simulink model "feedback_linearization_control"  (R2018b)
settings: Solver=VariableStepAuto  StartTime=0.0  StopTime=20  RelTol=1e-3
settings Model: Creator=Amirhossein  LastModifiedBy=Amirhossein

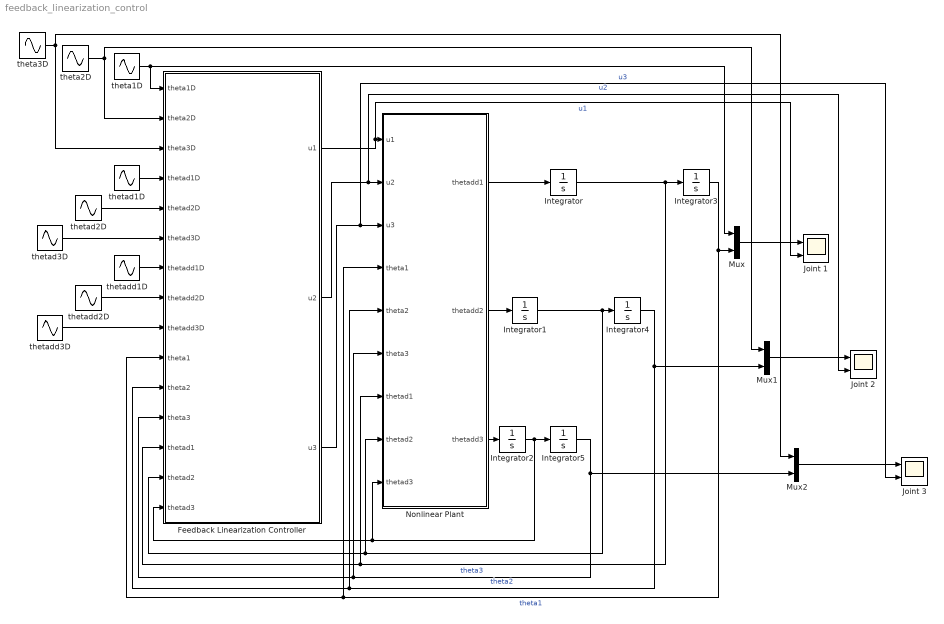
== system feedback_linearization_control ==
  Feedback Linearization Controller : MATLAB Function  TreatAsAtomicUnit=on
  Integrator{,1..5} (6 alike) : Integrator
  Joint 1 : Scope  NumInputPorts=2
  Joint 2 : Scope  NumInputPorts=2
  Joint 3 : Scope  NumInputPorts=2
  Mux : Mux  Inputs=2
  Mux1 : Mux  Inputs=2
  Mux2 : Mux  Inputs=2
  Nonlinear Plant : MATLAB Function  TreatAsAtomicUnit=on
  theta1D : Sin  SampleTime=0
  theta2D : Sin  Frequency=2  SampleTime=0
  theta3D : Sin  Frequency=3  SampleTime=0
  thetad1D : Sin  Phase=pi/2  SampleTime=0
  thetad2D : Sin  Amplitude=2  Frequency=2  Phase=pi/2  SampleTime=0
  thetad3D : Sin  Amplitude=3  Frequency=3  Phase=pi/2  SampleTime=0
  thetadd1D : Sin  Amplitude=-1  SampleTime=0
  thetadd2D : Sin  Amplitude=-4  Frequency=2  SampleTime=0
  thetadd3D : Sin  Amplitude=-9  Frequency=3  SampleTime=0
  wires:
  Integrator1/1 -> Integrator4/1, Feedback Linearization Controller/14(thetad2), Nonlinear Plant/8(thetad2)
  Integrator2/1 -> Feedback Linearization Controller/15(thetad3), Nonlinear Plant/9(thetad3), Integrator5/1
  Nonlinear Plant/1(thetadd1) -> Integrator/1
  Integrator/1 -> Feedback Linearization Controller/13(thetad1), Nonlinear Plant/7(thetad1), Integrator3/1
  Nonlinear Plant/2(thetadd2) -> Integrator1/1
  Nonlinear Plant/3(thetadd3) -> Integrator2/1
  Integrator3/1 -> Mux/2, Feedback Linearization Controller/10(theta1), Nonlinear Plant/4(theta1)  "theta1"
  Integrator4/1 -> Mux1/2, Feedback Linearization Controller/11(theta2), Nonlinear Plant/5(theta2)  "theta2"
  Feedback Linearization Controller/2(u2) -> Joint 2/2, Nonlinear Plant/2(u2)  "u2"
  Feedback Linearization Controller/1(u1) -> Joint 1/2, Nonlinear Plant/1(u1)  "u1"
  Feedback Linearization Controller/3(u3) -> Joint 3/2, Nonlinear Plant/3(u3)  "u3"
  Integrator5/1 -> Mux2/2, Feedback Linearization Controller/12(theta3), Nonlinear Plant/6(theta3)  "theta3"
  Mux1/1 -> Joint 2/1
  Mux2/1 -> Joint 3/1
  thetadd3D/1 -> Feedback Linearization Controller/9(thetadd3D)
  thetad1D/1 -> Feedback Linearization Controller/4(thetad1D)
  thetadd1D/1 -> Feedback Linearization Controller/7(thetadd1D)
  thetad3D/1 -> Feedback Linearization Controller/6(thetad3D)
  thetadd2D/1 -> Feedback Linearization Controller/8(thetadd2D)
  thetad2D/1 -> Feedback Linearization Controller/5(thetad2D)
  theta1D/1 -> Feedback Linearization Controller/1(theta1D), Mux/1
  theta2D/1 -> Mux1/1, Feedback Linearization Controller/2(theta2D)
  theta3D/1 -> Mux2/1, Feedback Linearization Controller/3(theta3D)
  Mux/1 -> Joint 1/1

== matlab function feedback_linearization_control/Feedback Linearization Controller ==
  data: theta1D input; theta2D input; u1 output; theta3D input; thetad1D input; thetad2D input; thetad3D input; thetadd1D input; thetadd2D input; thetadd3D input; theta1 input; theta2 input; theta3 input; thetad1 input; thetad2 input; thetad3 input; u2 output; u3 output
function [u1, u2, u3] = fcn(theta1D, theta2D, theta3D, thetad1D, thetad2D, thetad3D, thetadd1D, thetadd2D, thetadd3D, theta1, theta2, theta3, thetad1, thetad2, thetad3)

% lambda
lambda = 5;

thetaD = [theta1D; theta2D; theta3D];

thetadD = [thetad1D; thetad2D; thetad3D];

thetaddD = [thetadd1D; thetadd2D; thetadd3D];

% theta vector
theta = [theta1; theta2; theta3];

thetad = [thetad1; thetad2; thetad3];

e = theta - thetaD;

ed = thetad - thetadD;

%% model: the second model has been used

% the value of parameters
ma = 17.5e-3;
mc = 10.4e-3;
mbe = 0.2214;
mdf = 0.1106;
L1 = 13.97e-2;
L2 = 13.97e-2;
L3 = 0.325e-2;
L4 = 0.368e-2;
L5 = 0.527e-2;
g = 9.81;

% the elements of M matrix
m11 = ((0.5 * L1^2 + 0.125 * L2^2) * ma + (0.125 * L1^2 + 0.5 * L3^2) * mc) + 0.125 * L1^2 * (4*ma + mc) * cos(2*theta2) - 0.125 * (L2^2 * ma + 4 * L3^2 * mc) * cos(2*theta2) + 0.125 * (L2 * ma + L3 * mc) * cos(theta2) * sin(theta3);
m12 = 0;
m13 = 0;
m21 = m12;
m22 = L1^2 * (ma + 0.25 * mc);
m23 = -0.5 * L1 * (L2 * ma + L3 * mc) * sin(theta2 - theta3);
m31 = m13;
m32 = m23;
m33 = 0.25 * L2^2 * ma + L3^2 * mc;
% M matrix
M = [m11 m12 m13; m21 m22 m23; m31 m32 m33];

% the elements of V matrix
v11_1 = 0.25 * cos(theta3) * (2 * L1 * (L2 * ma + L3 * mc) * cos(theta2) + (L2^2 * ma + 4 * L3^2 * mc) * sin(theta3)) * thetad3;
v11 = 0.25 * (-2 * sin(theta2) * (L1^2 * (4 * ma + mc) * cos(theta2) + 2 * L1 * (L2 * ma + L3 * mc) * sin(theta3)) * thetad2) + v11_1;
v12 = -0.25 * (L1^2 * (4 * ma + mc) * sin(2 * theta2) + 2 * L1 * (L2 * ma + L3 * mc) * sin(theta2) * sin(theta3)) * thetad1;
v13 = -0.125 * (-4 * L1 * (L2 * ma + L3 * mc) * cos(theta2) * cos(theta3) - (L2^2 * ma + 4 * L3^2 * mc) * sin(2 * theta3)) * thetad1;
v21 = -v12;
v22 = 0;
v23 = 0.5 * L1 * (L2 * ma + L3 * mc) * cos(theta2 - theta3) * thetad3;
v31 = -v13;
v32 = 0.5 * L1 * (L2 * ma + L3 * mc) * cos(theta2 - theta3) * thetad2;
v33 = 0;
% V matrix
V = [v11 v12 v13; v21 v22 v23; v31 v32 v33];

% the elements of N vector
n1 = 0;
n2 = g * (L1 * (ma + 0.5 * mc) + L5 * mbe) * cos(theta2);
n3 = g * (0.5 * L2 * ma + L3 * mc - L4 * mdf ) * sin(theta3);
% N vector
N = [n1; n2; n3];

%%

W = thetaddD - 2 * lambda * ed - lambda^2 * e;

% U vector
U = M * W + V * thetad + N;

u1 = U(1);
u2 = U(2);
u3 = U(3);

== matlab function feedback_linearization_control/Nonlinear Plant ==
  data: u1 input; u2 input; thetadd1 output; u3 input; theta1 input; theta2 input; theta3 input; thetad1 input; thetad2 input; thetad3 input; thetadd2 output; thetadd3 output
function [thetadd1, thetadd2, thetadd3] = fcn(u1, u2, u3, theta1, theta2, theta3, thetad1, thetad2, thetad3)

% theta vector
thetad = [thetad1; thetad2; thetad3];

%% model: the second model has been used

% the value of parameters
ma = 17.5e-3;
mc = 10.4e-3;
mbe = 0.2214;
mdf = 0.1106;
L1 = 13.97e-2;
L2 = 13.97e-2;
L3 = 0.325e-2;
L4 = 0.368e-2;
L5 = 0.527e-2;
g = 9.81;

% the elements of M matrix
m11 = ((0.5 * L1^2 + 0.125 * L2^2) * ma + (0.125 * L1^2 + 0.5 * L3^2) * mc) + 0.125 * L1^2 * (4*ma + mc) * cos(2*theta2) - 0.125 * (L2^2 * ma + 4 * L3^2 * mc) * cos(2*theta2) + 0.125 * (L2 * ma + L3 * mc) * cos(theta2) * sin(theta3);
m12 = 0;
m13 = 0;
m21 = m12;
m22 = L1^2 * (ma + 0.25 * mc);
m23 = -0.5 * L1 * (L2 * ma + L3 * mc) * sin(theta2 - theta3);
m31 = m13;
m32 = m23;
m33 = 0.25 * L2^2 * ma + L3^2 * mc;
% M matrix
M = [m11 m12 m13; m21 m22 m23; m31 m32 m33];

% the elements of V matrix
v11_1 = 0.25 * cos(theta3) * (2 * L1 * (L2 * ma + L3 * mc) * cos(theta2) + (L2^2 * ma + 4 * L3^2 * mc) * sin(theta3)) * thetad3;
v11 = 0.25 * (-2 * sin(theta2) * (L1^2 * (4 * ma + mc) * cos(theta2) + 2 * L1 * (L2 * ma + L3 * mc) * sin(theta3)) * thetad2) + v11_1;
v12 = -0.25 * (L1^2 * (4 * ma + mc) * sin(2 * theta2) + 2 * L1 * (L2 * ma + L3 * mc) * sin(theta2) * sin(theta3)) * thetad1;
v13 = -0.125 * (-4 * L1 * (L2 * ma + L3 * mc) * cos(theta2) * cos(theta3) - (L2^2 * ma + 4 * L3^2 * mc) * sin(2 * theta3)) * thetad1;
v21 = -v12;
v22 = 0;
v23 = 0.5 * L1 * (L2 * ma + L3 * mc) * cos(theta2 - theta3) * thetad3;
v31 = -v13;
v32 = 0.5 * L1 * (L2 * ma + L3 * mc) * cos(theta2 - theta3) * thetad2;
v33 = 0;
% V matrix
V = [v11 v12 v13; v21 v22 v23; v31 v32 v33];

% the elements of N vector
n1 = 0;
n2 = g * (L1 * (ma + 0.5 * mc) + L5 * mbe) * cos(theta2);
n3 = g * (0.5 * L2 * ma + L3 * mc - L4 * mdf ) * sin(theta3);
% N vector
N = [n1; n2; n3];

%% 

% U vector
U = [u1; u2; u3];

B = V * thetad + N - U;

thetadd = - M \ B;

thetadd1 = thetadd(1);
thetadd2 = thetadd(2);
thetadd3 = thetadd(3);
